simulink model "mpc_OLD"  (R2021b)
settings: Solver=VariableStepAuto  StartTime=0.0  StopTime=10.0  RelTol=1e-3
libraries: mpclib x1, cstblocks x1
settings Model: Creator=emanu  LastModifiedBy=emanues
settings DebuggingCC: UnconnectedInputMsg=none  UnconnectedOutputMsg=none  UnconnectedLineMsg=none
settings ModelReferenceCC: EnableRefExpFcnMdlSchedulingChecks=off
settings RTWCC: DLArmComputeVersion=20.02.1

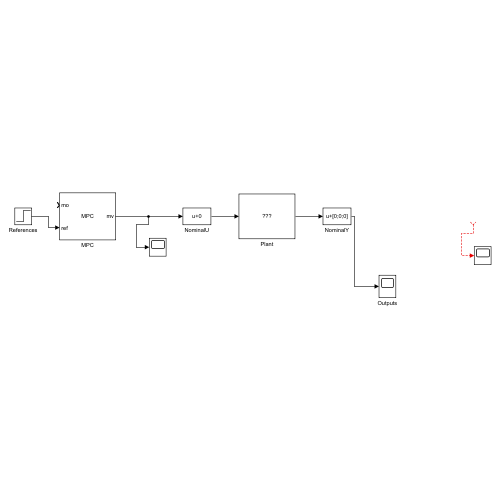
[thumbnail: Simulink's stored preview of the top-level diagram]
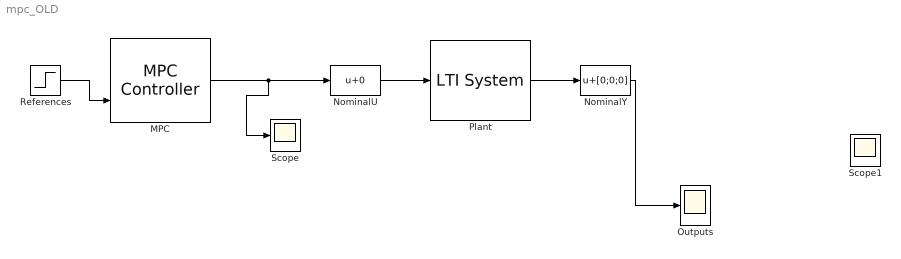
== system mpc_OLD ==
  MPC : mpclib/MPC Controller  SCDEnableBlockLinearizationSpecification=on  mpcobj=mpc1_C  is_multiple=0  enable_value=0  return_u0=off  updateMPCinCallerWorkspace=on  md_inport=off  mv_inport=off  uref_inport=off  return_cost=off  return_mvseq=off  return_qpstatus=off  return_xseq=off  return_state=off  return_ovseq=off  state_inport=off  umin_inport=off  umax_inport=off  ymin_inport=off  ymax_inport=off  cc_inport=off  ywt_inport=off  uwt_inport=off  duwt_inport=off  rhoeps_inport=off  pm_inport=off  MaximumP=10  HorizonChoice=FixedHorizon  n_ts=1  n_p=10  n_mv=1  n_md=0  n_ud=0  n_mo=3  n_uo=0  BlockDataType=double  SampleTimeInherited=off  switch_inport=off
  NominalU : Bias  SaturateOnIntegerOverflow=on
  NominalY : Bias  Bias=[0;0;0]  SaturateOnIntegerOverflow=on
  Outputs : Scope
  Plant : cstblocks/LTI System  sys=mpc1_G  IC=[]
  References : Step  Before=[0;0;0]  After=[1;1;1]
  Scope : Scope
  Scope1 : Scope
  wires:
  ? -> Scope1/1
  Plant/1 -> NominalY/1
  References/1 -> MPC/2
  NominalU/1 -> Plant/1
  MPC/1 -> Scope/1, NominalU/1
  NominalY/1 -> Outputs/1
